simulink library "Decoders_Lib"  (R2023a)
settings: Solver=ode45  StartTime=0.0  StopTime=10.0  RelTol=1e-3  EnableMultiTasking=on
(part 2 of 2)

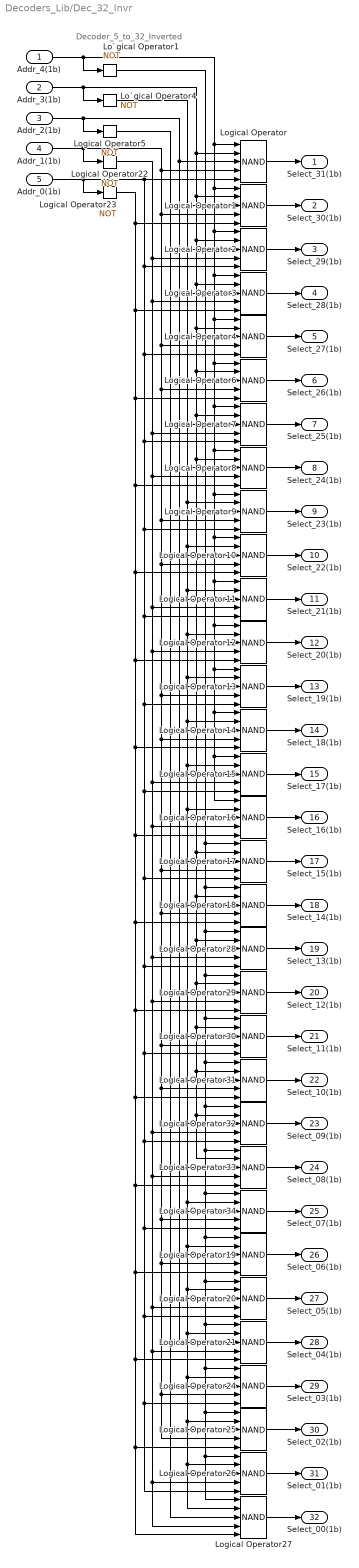
== system Decoders_Lib/Dec_32_Invr ==
  note: Decoder_5_to_32_Inverted
  Addr_4(1b) : Inport
  Addr_3(1b) : Inport  Port=2
  Addr_2(1b) : Inport  Port=3
  Addr_1(1b) : Inport  Port=4
  Addr_0(1b) : Inport  Port=5
  Lo`gical Operator1 : Logic  Operator=NOT  IconShape=distinctive  AllPortsSameDT=off  OutDataTypeStr=boolean
  Lo`gical Operator4 : Logic  Operator=NOT  IconShape=distinctive  AllPortsSameDT=off  OutDataTypeStr=boolean
  Logical Operator{,1..4,6..21,24..34} (32 alike) : Logic  Operator=NAND  Inputs=5  IconShape=distinctive  AllPortsSameDT=off  OutDataTypeStr=boolean
  Logical Operator22 : Logic  Operator=NOT  IconShape=distinctive  AllPortsSameDT=off  OutDataTypeStr=boolean
  Logical Operator23 : Logic  Operator=NOT  IconShape=distinctive  AllPortsSameDT=off  OutDataTypeStr=boolean
  Logical Operator5 : Logic  Operator=NOT  IconShape=distinctive  AllPortsSameDT=off  OutDataTypeStr=boolean
  Select_31(1b) : Outport
  Select_30(1b) : Outport  Port=2
  Select_29(1b) : Outport  Port=3
  Select_28(1b) : Outport  Port=4
  Select_27(1b) : Outport  Port=5
  Select_26(1b) : Outport  Port=6
  Select_25(1b) : Outport  Port=7
  Select_24(1b) : Outport  Port=8
  Select_23(1b) : Outport  Port=9
  Select_22(1b) : Outport  Port=10
  Select_21(1b) : Outport  Port=11
  Select_20(1b) : Outport  Port=12
  Select_19(1b) : Outport  Port=13
  Select_18(1b) : Outport  Port=14
  Select_17(1b) : Outport  Port=15
  Select_16(1b) : Outport  Port=16
  Select_15(1b) : Outport  Port=17
  Select_14(1b) : Outport  Port=18
  Select_13(1b) : Outport  Port=19
  Select_12(1b) : Outport  Port=20
  Select_11(1b) : Outport  Port=21
  Select_10(1b) : Outport  Port=22
  Select_09(1b) : Outport  Port=23
  Select_08(1b) : Outport  Port=24
  Select_07(1b) : Outport  Port=25
  Select_06(1b) : Outport  Port=26
  Select_05(1b) : Outport  Port=27
  Select_04(1b) : Outport  Port=28
  Select_03(1b) : Outport  Port=29
  Select_02(1b) : Outport  Port=30
  Select_01(1b) : Outport  Port=31
  Select_00(1b) : Outport  Port=32
  wires:
  Logical Operator16/1 -> Select_16(1b)/1
  Logical Operator15/1 -> Select_17(1b)/1
  Logical Operator14/1 -> Select_18(1b)/1
  Logical Operator13/1 -> Select_19(1b)/1
  Logical Operator12/1 -> Select_20(1b)/1
  Logical Operator11/1 -> Select_21(1b)/1
  Logical Operator10/1 -> Select_22(1b)/1
  Logical Operator9/1 -> Select_23(1b)/1
  Logical Operator8/1 -> Select_24(1b)/1
  Logical Operator7/1 -> Select_25(1b)/1
  Logical Operator6/1 -> Select_26(1b)/1
  Logical Operator4/1 -> Select_27(1b)/1
  Logical Operator1/1 -> Select_30(1b)/1
  Logical Operator2/1 -> Select_29(1b)/1
  Logical Operator3/1 -> Select_28(1b)/1
  Logical Operator/1 -> Select_31(1b)/1
  Logical Operator22/1 -> Logical Operator27/4, Logical Operator26/4, Logical Operator21/4, Logical Operator20/4, Logical Operator33/4, Logical Operator32/4, Logical Operator29/4, Logical Operator28/4, Logical Operator16/4, Logical Operator15/4, Logical Operator12/4, Logical Operator11/4, Logical Operator8/4, Logical Operator7/4, Logical Operator3/4, Logical Operator2/4
  Addr_0(1b)/1 -> Logical Operator26/5, Logical Operator24/5, Logical Operator20/5, Logical Operator34/5, Logical Operator32/5, Logical Operator30/5, Logical Operator28/5, Logical Operator17/5, Logical Operator15/5, Logical Operator13/5, Logical Operator11/5, Logical Operator9/5, Logical Operator7/5, Logical Operator4/5, Logical Operator2/5, Logical Operator/5, Logical Operator23/1
  Logical Operator23/1 -> Logical Operator27/5, Logical Operator25/5, Logical Operator21/5, Logical Operator19/5, Logical Operator33/5, Logical Operator31/5, Logical Operator29/5, Logical Operator18/5, Logical Operator16/5, Logical Operator14/5, Logical Operator12/5, Logical Operator10/5, Logical Operator8/5, Logical Operator6/5, Logical Operator3/5, Logical Operator1/5
  Logical Operator5/1 -> Logical Operator27/3, Logical Operator26/3, Logical Operator25/3, Logical Operator24/3, Logical Operator33/3, Logical Operator32/3, Logical Operator31/3, Logical Operator30/3, Logical Operator16/3, Logical Operator15/3, Logical Operator14/3, Logical Operator13/3, Logical Operator8/3, Logical Operator7/3, Logical Operator6/3, Logical Operator4/3
  Addr_3(1b)/1 -> Lo`gical Operator4/1, Logical Operator33/2, Logical Operator32/2, Logical Operator31/2, Logical Operator30/2, Logical Operator29/2, Logical Operator28/2, Logical Operator18/2, Logical Operator17/2, Logical Operator8/2, Logical Operator7/2, Logical Operator6/2, Logical Operator4/2, Logical Operator3/2, Logical Operator2/2, Logical Operator1/2, Logical Operator/2
  Addr_1(1b)/1 -> Logical Operator22/1, Logical Operator25/4, Logical Operator24/4, Logical Operator19/4, Logical Operator34/4, Logical Operator31/4, Logical Operator30/4, Logical Operator18/4, Logical Operator17/4, Logical Operator14/4, Logical Operator13/4, Logical Operator10/4, Logical Operator9/4, Logical Operator6/4, Logical Operator4/4, Logical Operator1/4, Logical Operator/4
  Addr_2(1b)/1 -> Logical Operator21/3, Logical Operator20/3, Logical Operator19/3, Logical Operator34/3, Logical Operator29/3, Logical Operator28/3, Logical Operator18/3, Logical Operator17/3, Logical Operator12/3, Logical Operator11/3, Logical Operator10/3, Logical Operator9/3, Logical Operator3/3, Logical Operator2/3, Logical Operator1/3, Logical Operator/3, Logical Operator5/1
  Lo`gical Operator4/1 -> Logical Operator27/2, Logical Operator26/2, Logical Operator25/2, Logical Operator24/2, Logical Operator21/2, Logical Operator20/2, Logical Operator19/2, Logical Operator34/2, Logical Operator16/2, Logical Operator15/2, Logical Operator14/2, Logical Operator13/2, Logical Operator12/2, Logical Operator11/2, Logical Operator10/2, Logical Operator9/2
  Logical Operator27/1 -> Select_00(1b)/1
  Logical Operator26/1 -> Select_01(1b)/1
  Logical Operator25/1 -> Select_02(1b)/1
  Logical Operator24/1 -> Select_03(1b)/1
  Logical Operator21/1 -> Select_04(1b)/1
  Logical Operator20/1 -> Select_05(1b)/1
  Logical Operator19/1 -> Select_06(1b)/1
  Logical Operator34/1 -> Select_07(1b)/1
  Logical Operator33/1 -> Select_08(1b)/1
  Logical Operator32/1 -> Select_09(1b)/1
  Logical Operator31/1 -> Select_10(1b)/1
  Logical Operator30/1 -> Select_11(1b)/1
  Logical Operator18/1 -> Select_14(1b)/1
  Logical Operator28/1 -> Select_13(1b)/1
  Logical Operator29/1 -> Select_12(1b)/1
  Logical Operator17/1 -> Select_15(1b)/1
  Lo`gical Operator1/1 -> Logical Operator27/1, Logical Operator26/1, Logical Operator25/1, Logical Operator24/1, Logical Operator21/1, Logical Operator20/1, Logical Operator19/1, Logical Operator34/1, Logical Operator33/1, Logical Operator32/1, Logical Operator31/1, Logical Operator30/1, Logical Operator29/1, Logical Operator28/1, Logical Operator18/1, Logical Operator17/1
  Addr_4(1b)/1 -> Logical Operator16/1, Logical Operator15/1, Logical Operator14/1, Logical Operator13/1, Logical Operator12/1, Logical Operator11/1, Logical Operator10/1, Logical Operator9/1, Logical Operator8/1, Logical Operator7/1, Logical Operator6/1, Logical Operator4/1, Logical Operator3/1, Logical Operator2/1, Logical Operator1/1, Logical Operator/1, Lo`gical Operator1/1

== system Decoders_Lib/Dec_4 ==
  note: Decoder_2_to_4
  Addr_1(1b) : Inport
  Addr_0(1b) : Inport  Port=2
  Logical Operator{1..4,22..23} (6 alike) : Logic  Operator=NOT  IconShape=distinctive  AllPortsSameDT=off  OutDataTypeStr=boolean
  Logical Operator{14..17} (4 alike) : Logic  Operator=NAND  IconShape=distinctive  AllPortsSameDT=off  OutDataTypeStr=boolean
  Select_3(1b) : Outport
  Select_2(1b) : Outport  Port=2
  Select_1(1b) : Outport  Port=3
  Select_0(1b) : Outport  Port=4
  wires:
  Logical Operator14/1 -> Logical Operator4/1
  Logical Operator15/1 -> Logical Operator3/1
  Logical Operator16/1 -> Logical Operator2/1
  Logical Operator17/1 -> Logical Operator1/1
  Addr_1(1b)/1 -> Logical Operator22/1, Logical Operator15/1, Logical Operator14/1
  Logical Operator23/1 -> Logical Operator15/2, Logical Operator17/2
  Logical Operator22/1 -> Logical Operator16/1, Logical Operator17/1
  Addr_0(1b)/1 -> Logical Operator14/2, Logical Operator16/2, Logical Operator23/1
  Logical Operator1/1 -> Select_0(1b)/1
  Logical Operator2/1 -> Select_1(1b)/1
  Logical Operator3/1 -> Select_2(1b)/1
  Logical Operator4/1 -> Select_3(1b)/1

== system Decoders_Lib/Dec_4_Enbl ==
  note: Decoder_2_to_4_Enabled
  Enable(1b) : Inport
  Addr_1(1b) : Inport  Port=2
  Addr_0(1b) : Inport  Port=3
  Logical Operator{1..4,22..23} (6 alike) : Logic  Operator=NOT  IconShape=distinctive  AllPortsSameDT=off  OutDataTypeStr=boolean
  Logical Operator{14..17} (4 alike) : Logic  Operator=NAND  Inputs=3  IconShape=distinctive  AllPortsSameDT=off  OutDataTypeStr=boolean
  Select_3(1b) : Outport
  Select_2(1b) : Outport  Port=2
  Select_1(1b) : Outport  Port=3
  Select_0(1b) : Outport  Port=4
  wires:
  Enable(1b)/1 -> Logical Operator17/1, Logical Operator16/1, Logical Operator15/1, Logical Operator14/1
  Logical Operator14/1 -> Logical Operator4/1
  Logical Operator15/1 -> Logical Operator3/1
  Logical Operator16/1 -> Logical Operator2/1
  Logical Operator17/1 -> Logical Operator1/1
  Addr_1(1b)/1 -> Logical Operator22/1, Logical Operator14/2, Logical Operator15/2
  Logical Operator23/1 -> Logical Operator15/3, Logical Operator17/3
  Logical Operator22/1 -> Logical Operator16/2, Logical Operator17/2
  Addr_0(1b)/1 -> Logical Operator23/1, Logical Operator14/3, Logical Operator16/3
  Logical Operator1/1 -> Select_0(1b)/1
  Logical Operator2/1 -> Select_1(1b)/1
  Logical Operator3/1 -> Select_2(1b)/1
  Logical Operator4/1 -> Select_3(1b)/1

== system Decoders_Lib/Dec_4_Enbl_Invr ==
  note: Decoder_2_to_4_Enabled_Inverting
  Enable(1b) : Inport
  Addr_1(1b) : Inport  Port=2
  Addr_0(1b) : Inport  Port=3
  Logical Operator{14..17} (4 alike) : Logic  Operator=NAND  Inputs=3  IconShape=distinctive  AllPortsSameDT=off  OutDataTypeStr=boolean
  Logical Operator22 : Logic  Operator=NOT  IconShape=distinctive  AllPortsSameDT=off  OutDataTypeStr=boolean
  Logical Operator23 : Logic  Operator=NOT  IconShape=distinctive  AllPortsSameDT=off  OutDataTypeStr=boolean
  Select_3(1b) : Outport
  Select_2(1b) : Outport  Port=2
  Select_1(1b) : Outport  Port=3
  Select_0(1b) : Outport  Port=4
  wires:
  Enable(1b)/1 -> Logical Operator17/1, Logical Operator16/1, Logical Operator15/1, Logical Operator14/1
  Logical Operator14/1 -> Select_3(1b)/1
  Logical Operator15/1 -> Select_2(1b)/1
  Logical Operator16/1 -> Select_1(1b)/1
  Logical Operator17/1 -> Select_0(1b)/1
  Addr_1(1b)/1 -> Logical Operator22/1, Logical Operator14/2, Logical Operator15/2
  Logical Operator23/1 -> Logical Operator15/3, Logical Operator17/3
  Logical Operator22/1 -> Logical Operator16/2, Logical Operator17/2
  Addr_0(1b)/1 -> Logical Operator23/1, Logical Operator14/3, Logical Operator16/3

== system Decoders_Lib/Dec_4_Invr ==
  note: Decoder_2_to_4_Inverting
  Addr_1(1b) : Inport
  Addr_0(1b) : Inport  Port=2
  Logical Operator{14..17} (4 alike) : Logic  Operator=NAND  IconShape=distinctive  AllPortsSameDT=off  OutDataTypeStr=boolean
  Logical Operator22 : Logic  Operator=NOT  IconShape=distinctive  AllPortsSameDT=off  OutDataTypeStr=boolean
  Logical Operator23 : Logic  Operator=NOT  IconShape=distinctive  AllPortsSameDT=off  OutDataTypeStr=boolean
  Select_3(1b) : Outport
  Select_2(1b) : Outport  Port=2
  Select_1(1b) : Outport  Port=3
  Select_0(1b) : Outport  Port=4
  wires:
  Addr_1(1b)/1 -> Logical Operator22/1, Logical Operator15/1, Logical Operator14/1
  Logical Operator23/1 -> Logical Operator15/2, Logical Operator17/2
  Logical Operator22/1 -> Logical Operator16/1, Logical Operator17/1
  Addr_0(1b)/1 -> Logical Operator14/2, Logical Operator16/2, Logical Operator23/1
  Logical Operator17/1 -> Select_0(1b)/1
  Logical Operator16/1 -> Select_1(1b)/1
  Logical Operator15/1 -> Select_2(1b)/1
  Logical Operator14/1 -> Select_3(1b)/1

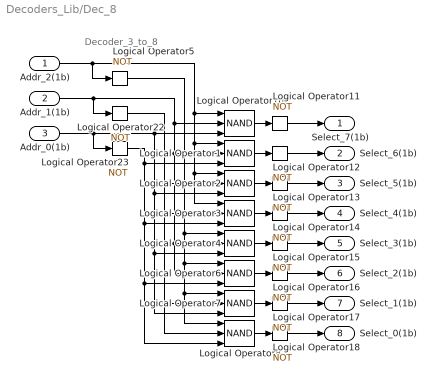
== system Decoders_Lib/Dec_8 ==
  note: Decoder_3_to_8
  Addr_2(1b) : Inport
  Addr_1(1b) : Inport  Port=2
  Addr_0(1b) : Inport  Port=3
  Logical Operator{1..4,6..8,10} (8 alike) : Logic  Operator=NAND  Inputs=3  IconShape=distinctive  AllPortsSameDT=off  OutDataTypeStr=boolean
  Logical Operator{5,11..18,22..23} (11 alike) : Logic  Operator=NOT  IconShape=distinctive  AllPortsSameDT=off  OutDataTypeStr=boolean
  Select_7(1b) : Outport
  Select_6(1b) : Outport  Port=2
  Select_5(1b) : Outport  Port=3
  Select_4(1b) : Outport  Port=4
  Select_3(1b) : Outport  Port=5
  Select_2(1b) : Outport  Port=6
  Select_1(1b) : Outport  Port=7
  Select_0(1b) : Outport  Port=8
  wires:
  Addr_0(1b)/1 -> Logical Operator10/3, Logical Operator7/3, Logical Operator4/3, Logical Operator2/3, Logical Operator23/1
  Logical Operator22/1 -> Logical Operator8/2, Logical Operator7/2, Logical Operator3/2, Logical Operator2/2
  Logical Operator23/1 -> Logical Operator8/3, Logical Operator6/3, Logical Operator3/3, Logical Operator1/3
  Addr_2(1b)/1 -> Logical Operator10/1, Logical Operator3/1, Logical Operator2/1, Logical Operator1/1, Logical Operator5/1
  Addr_1(1b)/1 -> Logical Operator10/2, Logical Operator1/2, Logical Operator6/2, Logical Operator4/2, Logical Operator22/1
  Logical Operator8/1 -> Logical Operator18/1
  Logical Operator7/1 -> Logical Operator17/1
  Logical Operator6/1 -> Logical Operator16/1
  Logical Operator4/1 -> Logical Operator15/1
  Logical Operator3/1 -> Logical Operator14/1
  Logical Operator2/1 -> Logical Operator13/1
  Logical Operator1/1 -> Logical Operator12/1
  Logical Operator10/1 -> Logical Operator11/1
  Logical Operator5/1 -> Logical Operator8/1, Logical Operator7/1, Logical Operator6/1, Logical Operator4/1
  Logical Operator11/1 -> Select_7(1b)/1
  Logical Operator12/1 -> Select_6(1b)/1
  Logical Operator13/1 -> Select_5(1b)/1
  Logical Operator14/1 -> Select_4(1b)/1
  Logical Operator15/1 -> Select_3(1b)/1
  Logical Operator16/1 -> Select_2(1b)/1
  Logical Operator17/1 -> Select_1(1b)/1
  Logical Operator18/1 -> Select_0(1b)/1

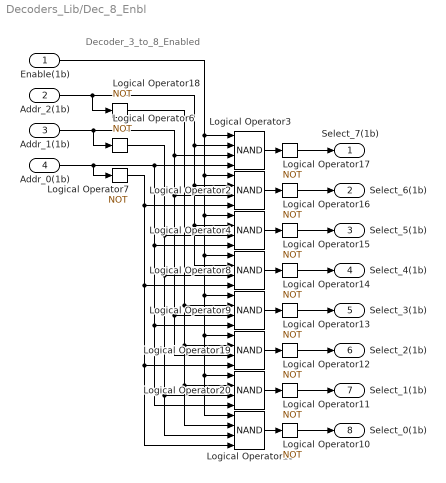
== system Decoders_Lib/Dec_8_Enbl ==
  note: Decoder_3_to_8_Enabled
  Enable(1b) : Inport
  Addr_2(1b) : Inport  Port=2
  Addr_1(1b) : Inport  Port=3
  Addr_0(1b) : Inport  Port=4
  Logical Operator{6..7,10..18} (11 alike) : Logic  Operator=NOT  IconShape=distinctive  AllPortsSameDT=off  OutDataTypeStr=boolean
  Logical Operator{2..4,8..9,19..20,25} (8 alike) : Logic  Operator=NAND  Inputs=4  IconShape=distinctive  AllPortsSameDT=off  OutDataTypeStr=boolean
  Select_7(1b) : Outport
  Select_6(1b) : Outport  Port=2
  Select_5(1b) : Outport  Port=3
  Select_4(1b) : Outport  Port=4
  Select_3(1b) : Outport  Port=5
  Select_2(1b) : Outport  Port=6
  Select_1(1b) : Outport  Port=7
  Select_0(1b) : Outport  Port=8
  wires:
  Logical Operator2/1 -> Logical Operator16/1
  Logical Operator20/1 -> Logical Operator11/1
  Addr_1(1b)/1 -> Logical Operator3/3, Logical Operator2/3, Logical Operator9/3, Logical Operator19/3, Logical Operator6/1
  Logical Operator3/1 -> Logical Operator17/1
  Logical Operator8/1 -> Logical Operator14/1
  Logical Operator9/1 -> Logical Operator13/1
  Addr_2(1b)/1 -> Logical Operator3/2, Logical Operator2/2, Logical Operator4/2, Logical Operator8/2, Logical Operator18/1
  Logical Operator25/1 -> Logical Operator10/1
  Logical Operator19/1 -> Logical Operator12/1
  Logical Operator6/1 -> Logical Operator4/3, Logical Operator8/3, Logical Operator20/3, Logical Operator25/3
  Logical Operator4/1 -> Logical Operator15/1
  Addr_0(1b)/1 -> Logical Operator3/4, Logical Operator4/4, Logical Operator9/4, Logical Operator20/4, Logical Operator7/1
  Logical Operator18/1 -> Logical Operator9/2, Logical Operator19/2, Logical Operator20/2, Logical Operator25/2
  Logical Operator7/1 -> Logical Operator2/4, Logical Operator8/4, Logical Operator19/4, Logical Operator25/4
  Enable(1b)/1 -> Logical Operator19/1, Logical Operator20/1, Logical Operator25/1, Logical Operator9/1, Logical Operator8/1, Logical Operator4/1, Logical Operator2/1, Logical Operator3/1
  Logical Operator10/1 -> Select_0(1b)/1
  Logical Operator11/1 -> Select_1(1b)/1
  Logical Operator12/1 -> Select_2(1b)/1
  Logical Operator13/1 -> Select_3(1b)/1
  Logical Operator14/1 -> Select_4(1b)/1
  Logical Operator15/1 -> Select_5(1b)/1
  Logical Operator16/1 -> Select_6(1b)/1
  Logical Operator17/1 -> Select_7(1b)/1

== system Decoders_Lib/Dec_8_Enbl_Invr ==
  note: Decoder_3_to_8_Enabled_Inverting
  Enable(1b) : Inport
  Addr_2(1b) : Inport  Port=2
  Addr_1(1b) : Inport  Port=3
  Addr_0(1b) : Inport  Port=4
  Logical Operator18 : Logic  Operator=NOT  IconShape=distinctive  AllPortsSameDT=off  OutDataTypeStr=boolean
  Logical Operator{2..4,8..9,19..20,25} (8 alike) : Logic  Operator=NAND  Inputs=4  IconShape=distinctive  AllPortsSameDT=off  OutDataTypeStr=boolean
  Logical Operator6 : Logic  Operator=NOT  IconShape=distinctive  AllPortsSameDT=off  OutDataTypeStr=boolean
  Logical Operator7 : Logic  Operator=NOT  IconShape=distinctive  AllPortsSameDT=off  OutDataTypeStr=boolean
  Select_7(1b) : Outport
  Select_6(1b) : Outport  Port=2
  Select_5(1b) : Outport  Port=3
  Select_4(1b) : Outport  Port=4
  Select_3(1b) : Outport  Port=5
  Select_2(1b) : Outport  Port=6
  Select_1(1b) : Outport  Port=7
  Select_0(1b) : Outport  Port=8
  wires:
  Logical Operator2/1 -> Select_6(1b)/1
  Logical Operator20/1 -> Select_1(1b)/1
  Addr_1(1b)/1 -> Logical Operator3/3, Logical Operator2/3, Logical Operator9/3, Logical Operator19/3, Logical Operator6/1
  Logical Operator3/1 -> Select_7(1b)/1
  Logical Operator8/1 -> Select_4(1b)/1
  Logical Operator9/1 -> Select_3(1b)/1
  Addr_2(1b)/1 -> Logical Operator3/2, Logical Operator2/2, Logical Operator4/2, Logical Operator8/2, Logical Operator18/1
  Logical Operator25/1 -> Select_0(1b)/1
  Logical Operator19/1 -> Select_2(1b)/1
  Logical Operator6/1 -> Logical Operator4/3, Logical Operator8/3, Logical Operator20/3, Logical Operator25/3
  Logical Operator4/1 -> Select_5(1b)/1
  Addr_0(1b)/1 -> Logical Operator3/4, Logical Operator4/4, Logical Operator9/4, Logical Operator20/4, Logical Operator7/1
  Logical Operator18/1 -> Logical Operator9/2, Logical Operator19/2, Logical Operator20/2, Logical Operator25/2
  Logical Operator7/1 -> Logical Operator2/4, Logical Operator8/4, Logical Operator19/4, Logical Operator25/4
  Enable(1b)/1 -> Logical Operator19/1, Logical Operator20/1, Logical Operator25/1, Logical Operator9/1, Logical Operator8/1, Logical Operator4/1, Logical Operator2/1, Logical Operator3/1

== system Decoders_Lib/Dec_8_Invr ==
  note: Decoder_3_to_8_Inverting
  Addr_2(1b) : Inport
  Addr_1(1b) : Inport  Port=2
  Addr_0(1b) : Inport  Port=3
  Logical Operator{1..4,6..8,10} (8 alike) : Logic  Operator=NAND  Inputs=3  IconShape=distinctive  AllPortsSameDT=off  OutDataTypeStr=boolean
  Logical Operator22 : Logic  Operator=NOT  IconShape=distinctive  AllPortsSameDT=off  OutDataTypeStr=boolean
  Logical Operator23 : Logic  Operator=NOT  IconShape=distinctive  AllPortsSameDT=off  OutDataTypeStr=boolean
  Logical Operator5 : Logic  Operator=NOT  IconShape=distinctive  AllPortsSameDT=off  OutDataTypeStr=boolean
  Select_7(1b) : Outport
  Select_6(1b) : Outport  Port=2
  Select_5(1b) : Outport  Port=3
  Select_4(1b) : Outport  Port=4
  Select_3(1b) : Outport  Port=5
  Select_2(1b) : Outport  Port=6
  Select_1(1b) : Outport  Port=7
  Select_0(1b) : Outport  Port=8
  wires:
  Addr_0(1b)/1 -> Logical Operator10/3, Logical Operator7/3, Logical Operator4/3, Logical Operator2/3, Logical Operator23/1
  Logical Operator22/1 -> Logical Operator8/2, Logical Operator7/2, Logical Operator3/2, Logical Operator2/2
  Logical Operator23/1 -> Logical Operator8/3, Logical Operator6/3, Logical Operator3/3, Logical Operator1/3
  Addr_2(1b)/1 -> Logical Operator10/1, Logical Operator3/1, Logical Operator2/1, Logical Operator1/1, Logical Operator5/1
  Addr_1(1b)/1 -> Logical Operator10/2, Logical Operator1/2, Logical Operator6/2, Logical Operator4/2, Logical Operator22/1
  Logical Operator8/1 -> Select_0(1b)/1
  Logical Operator7/1 -> Select_1(1b)/1
  Logical Operator6/1 -> Select_2(1b)/1
  Logical Operator4/1 -> Select_3(1b)/1
  Logical Operator3/1 -> Select_4(1b)/1
  Logical Operator2/1 -> Select_5(1b)/1
  Logical Operator1/1 -> Select_6(1b)/1
  Logical Operator10/1 -> Select_7(1b)/1
  Logical Operator5/1 -> Logical Operator8/1, Logical Operator7/1, Logical Operator6/1, Logical Operator4/1

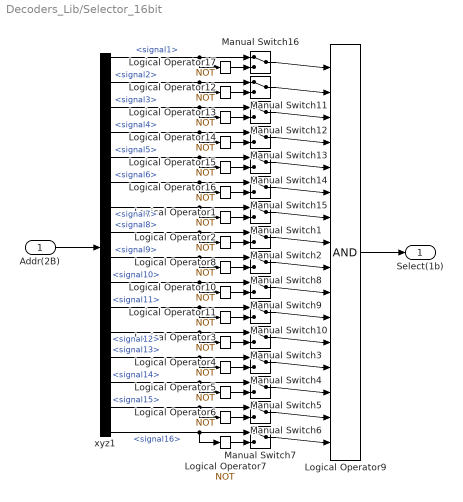
== system Decoders_Lib/Selector_16bit ==
  Addr(2B) : Inport
  Logical Operator{1..8,10..17} (16 alike) : Logic  Operator=NOT  Inputs=1  IconShape=distinctive  AllPortsSameDT=off  OutDataTypeStr=boolean
  Logical Operator9 : Logic  Inputs=16  IconShape=distinctive  AllPortsSameDT=off  OutDataTypeStr=boolean
  Manual Switch{1..16} (16 alike) : ManualSwitch
  xyz1 : BusSelector  OutputSignals=signal1,signal2,signal3,signal4,signal5,signal6,signal7,signal8,signal9,signal10,signal11,signal12,signal13,signal14,signal15,signal16
  Select(1b) : Outport
  wires:
  Addr(2B)/1 -> xyz1/1
  Logical Operator9/1 -> Select(1b)/1
  Manual Switch3/1 -> Logical Operator9/12
  xyz1/12 -> Logical Operator3/1, Manual Switch3/1  "<signal12>"
  Manual Switch4/1 -> Logical Operator9/13
  xyz1/13 -> Logical Operator4/1, Manual Switch4/1  "<signal13>"
  Manual Switch5/1 -> Logical Operator9/14
  xyz1/14 -> Logical Operator5/1, Manual Switch5/1  "<signal14>"
  Manual Switch6/1 -> Logical Operator9/15
  xyz1/15 -> Logical Operator6/1, Manual Switch6/1  "<signal15>"
  Manual Switch7/1 -> Logical Operator9/16
  xyz1/16 -> Logical Operator7/1, Manual Switch7/1  "<signal16>"
  Logical Operator3/1 -> Manual Switch3/2
  Logical Operator7/1 -> Manual Switch7/2
  Logical Operator6/1 -> Manual Switch6/2
  Logical Operator5/1 -> Manual Switch5/2
  Logical Operator4/1 -> Manual Switch4/2
  Manual Switch1/1 -> Logical Operator9/7
  xyz1/7 -> Logical Operator1/1, Manual Switch1/1  "<signal7>"
  Manual Switch2/1 -> Logical Operator9/8
  xyz1/8 -> Logical Operator2/1, Manual Switch2/1  "<signal8>"
  Manual Switch8/1 -> Logical Operator9/9
  xyz1/9 -> Logical Operator8/1, Manual Switch8/1  "<signal9>"
  Manual Switch9/1 -> Logical Operator9/10
  xyz1/10 -> Logical Operator10/1, Manual Switch9/1  "<signal10>"
  Manual Switch10/1 -> Logical Operator9/11
  xyz1/11 -> Logical Operator11/1, Manual Switch10/1  "<signal11>"
  Logical Operator1/1 -> Manual Switch1/2
  Logical Operator11/1 -> Manual Switch10/2
  Logical Operator10/1 -> Manual Switch9/2
  Logical Operator8/1 -> Manual Switch8/2
  Logical Operator2/1 -> Manual Switch2/2
  Manual Switch11/1 -> Logical Operator9/2
  xyz1/2 -> Logical Operator12/1, Manual Switch11/1  "<signal2>"
  Manual Switch12/1 -> Logical Operator9/3
  xyz1/3 -> Logical Operator13/1, Manual Switch12/1  "<signal3>"
  Manual Switch13/1 -> Logical Operator9/4
  xyz1/4 -> Logical Operator14/1, Manual Switch13/1  "<signal4>"
  Manual Switch14/1 -> Logical Operator9/5
  xyz1/5 -> Logical Operator15/1, Manual Switch14/1  "<signal5>"
  Manual Switch15/1 -> Logical Operator9/6
  xyz1/6 -> Logical Operator16/1, Manual Switch15/1  "<signal6>"
  Logical Operator12/1 -> Manual Switch11/2
  Logical Operator16/1 -> Manual Switch15/2
  Logical Operator15/1 -> Manual Switch14/2
  Logical Operator14/1 -> Manual Switch13/2
  Logical Operator13/1 -> Manual Switch12/2
  Manual Switch16/1 -> Logical Operator9/1
  xyz1/1 -> Logical Operator17/1, Manual Switch16/1  "<signal1>"
  Logical Operator17/1 -> Manual Switch16/2

== system Decoders_Lib/Selector_5bit ==
  Addr(1B) : Inport
  Bus Selector : BusSelector  OutputSignals=signal4,signal5,signal6,signal7,signal8
  Logical Operator{3..7} (5 alike) : Logic  Operator=NOT  Inputs=1  IconShape=distinctive  AllPortsSameDT=off  OutDataTypeStr=boolean
  Logical Operator9 : Logic  Inputs=5  IconShape=distinctive  AllPortsSameDT=off  OutDataTypeStr=boolean
  Manual Switch{3..7} (5 alike) : ManualSwitch
  Select(1b) : Outport
  wires:
  Addr(1B)/1 -> Bus Selector/1
  Logical Operator9/1 -> Select(1b)/1
  Manual Switch3/1 -> Logical Operator9/1
  Bus Selector/1 -> Logical Operator3/1, Manual Switch3/1  "<signal4>"
  Manual Switch4/1 -> Logical Operator9/2
  Bus Selector/2 -> Logical Operator4/1, Manual Switch4/1  "<signal5>"
  Manual Switch5/1 -> Logical Operator9/3
  Bus Selector/3 -> Logical Operator5/1, Manual Switch5/1  "<signal6>"
  Manual Switch6/1 -> Logical Operator9/4
  Bus Selector/4 -> Logical Operator6/1, Manual Switch6/1  "<signal7>"
  Manual Switch7/1 -> Logical Operator9/5
  Bus Selector/5 -> Logical Operator7/1, Manual Switch7/1  "<signal8>"
  Logical Operator3/1 -> Manual Switch3/2
  Logical Operator7/1 -> Manual Switch7/2
  Logical Operator6/1 -> Manual Switch6/2
  Logical Operator5/1 -> Manual Switch5/2
  Logical Operator4/1 -> Manual Switch4/2
